simulink model "filterbank"  (R2018a)
settings: Solver=FixedStepDiscrete  StartTime=0.0  StopTime=inf  RelTol=1e-3
libraries: audiofilters x16, dspsrcs4 x2
settings Model: Creator=Kavi  LastModifiedBy=Kavi
settings SolverCC: AutoInsertRateTranBlk=on
settings DataIOCC: LimitDataPoints=on  SaveOutput=off  SignalLogging=off  SaveTime=off
settings OptimizationCC: LifeSpan=inf  SimCompilerOptimization=on
settings DebuggingCC: AlgebraicLoopMsg=error  SingleTaskRateTransMsg=error  AllowSymbolicDim=off  SFUnexpectedBacktrackingDiag=warning  SFNoUnconditionalDefaultTransitionDiag=warning  SFExecutionAtInitializationDiag=none
settings CodeAppCC: StateflowObjectComments=on
settings GRTTargetCC: TargetLangStandard=C89/C90 (ANSI)  GeneratePreprocessorConditionals=Disable all
settings ConfigComp: CovMetricSettings=dw  CovHtmlReporting=on  CovSaveCumulativeToWorkspaceVar=on  CovSaveSingleToWorkspaceVar=on  CovExternalEMLEnable=off  CovSFcnEnable=off

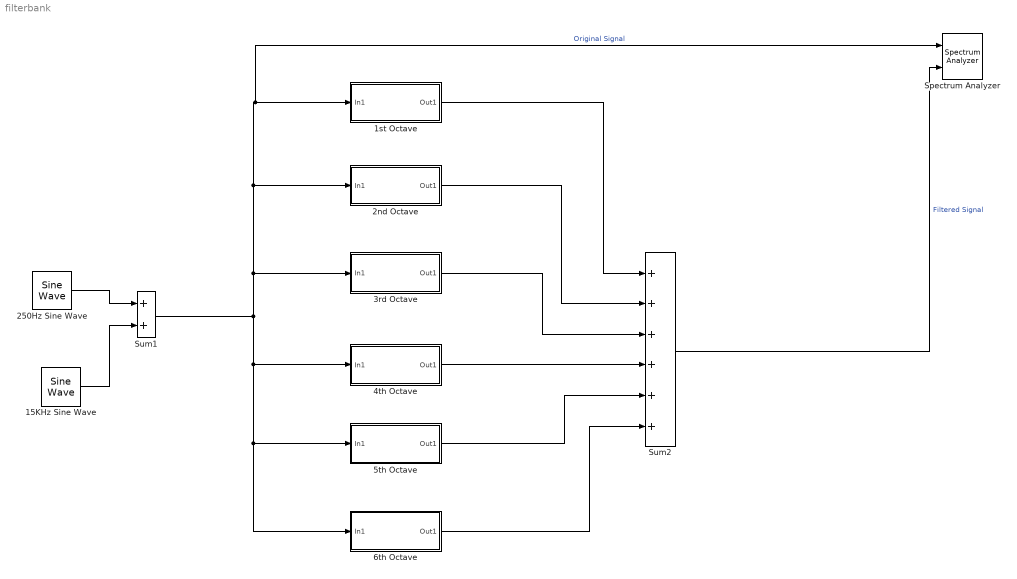
== system filterbank ==
  15KHz Sine Wave : dspsrcs4/Sine Wave  Amplitude=1  Frequency=314.98  Phase=0  SampleMode=Discrete  OutComplex=Real  CompMethod=Trigonometric fcn  TableSize=Speed  SampleTime=1/44100  SamplesPerFrame=256  ResetState=Restart at time zero  OutputFrames=off  dataType=double  wordLen=16  udDataType=sfix(16)  fracBitsMode=Best precision  numFracBits=15  OutDataTypeStr=double  LastOutDataTypeStr=double
  "1st Octave " : Subsystem
  250Hz Sine Wave : dspsrcs4/Sine Wave  Amplitude=1  Frequency=250  Phase=0  SampleMode=Discrete  OutComplex=Real  CompMethod=Trigonometric fcn  TableSize=Speed  SampleTime=1/44100  SamplesPerFrame=256  ResetState=Restart at time zero  OutputFrames=off  dataType=double  wordLen=16  udDataType=sfix(16)  fracBitsMode=Best precision  numFracBits=15  OutDataTypeStr=double  LastOutDataTypeStr=double
  2nd Octave : Subsystem
  "3rd Octave " : Subsystem
  4th Octave : Subsystem
  5th Octave : Subsystem
  6th Octave : Subsystem
  Spectrum Analyzer : SpectrumAnalyzer  NumInputPorts=2
  Sum1 : Sum
  Sum2 : Sum  Inputs=++++++
  wires:
  250Hz Sine Wave/1 -> Sum1/1
  15KHz Sine Wave/1 -> Sum1/2
  Sum1/1 -> "3rd Octave "/1(In1), "1st Octave "/1(In1), Spectrum Analyzer/1, 2nd Octave/1(In1), 6th Octave/1(In1), 5th Octave/1(In1), 4th Octave/1(In1)  "Original Signal"
  Sum2/1 -> Spectrum Analyzer/2  "Filtered Signal"
  2nd Octave/1(Out1) -> Sum2/2
  "3rd Octave "/1(Out1) -> Sum2/3
  4th Octave/1(Out1) -> Sum2/4
  5th Octave/1(Out1) -> Sum2/5
  6th Octave/1(Out1) -> Sum2/6
  "1st Octave "/1(Out1) -> Sum2/1

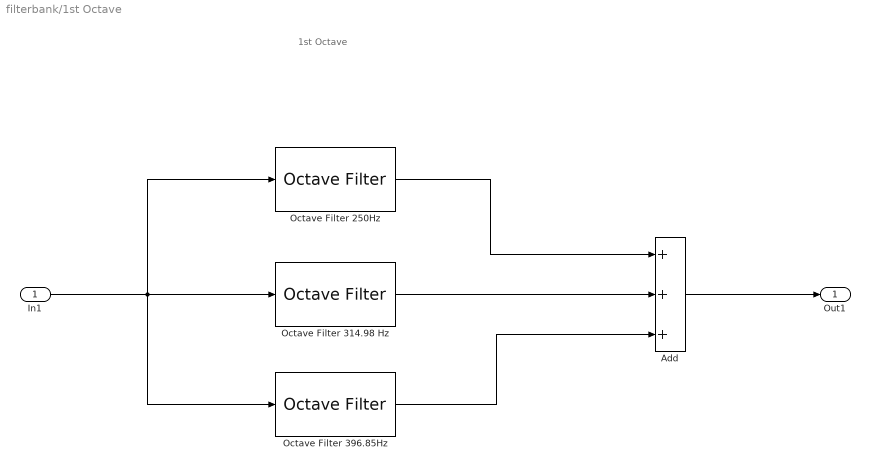
== system filterbank/1st Octave  ==
  note: 1st Octave
  In1 : Inport
  Add : Sum  Inputs=+++
  "Octave Filter 250Hz " : audiofilters/Octave Filter  FilterOrder=6  CenterFrequencyPort=off  CenterFrequency=250  Bandwidth=1 octave  BandsPerOctave=3  BandwidthType=1/3 octave  Oversample=off  InheritSampleRate=off  SampleRate=44100  SimulateUsing=Code generation  MaskClassType=Class 0
      settings: SourceProductName=Audio System Toolbox  SourceProductBaseCode=AU
  "Octave Filter 314.98 Hz " : audiofilters/Octave Filter  FilterOrder=6  CenterFrequencyPort=off  CenterFrequency=314.98  Bandwidth=1 octave  BandsPerOctave=3  BandwidthType=1/3 octave  Oversample=off  InheritSampleRate=off  SampleRate=44100  SimulateUsing=Code generation  MaskClassType=Class 0
      settings: SourceProductName=Audio System Toolbox  SourceProductBaseCode=AU
  "Octave Filter 396.85Hz " : audiofilters/Octave Filter  FilterOrder=6  CenterFrequencyPort=off  CenterFrequency=396.85  Bandwidth=1 octave  BandsPerOctave=3  BandwidthType=1/3 octave  Oversample=off  InheritSampleRate=off  SampleRate=44100  SimulateUsing=Code generation  MaskClassType=Class 0
      settings: SourceProductName=Audio System Toolbox  SourceProductBaseCode=AU
  Out1 : Outport
  wires:
  In1/1 -> "Octave Filter 250Hz "/1, "Octave Filter 314.98 Hz "/1, "Octave Filter 396.85Hz "/1
  "Octave Filter 314.98 Hz "/1 -> Add/2
  "Octave Filter 250Hz "/1 -> Add/1
  "Octave Filter 396.85Hz "/1 -> Add/3
  Add/1 -> Out1/1

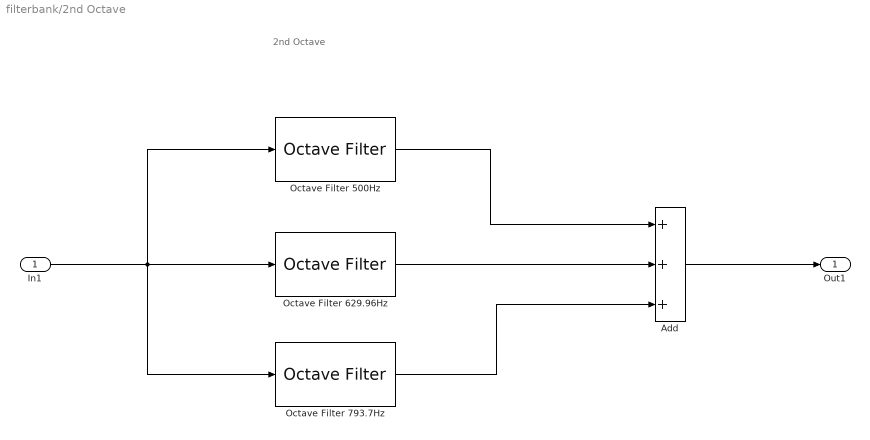
== system filterbank/2nd Octave ==
  note: 2nd Octave
  In1 : Inport
  Add : Sum  Inputs=+++
  "Octave Filter 500Hz " : audiofilters/Octave Filter  FilterOrder=6  CenterFrequencyPort=off  CenterFrequency=500  Bandwidth=1 octave  BandsPerOctave=3  BandwidthType=1/3 octave  Oversample=off  InheritSampleRate=off  SampleRate=44100  SimulateUsing=Code generation  MaskClassType=Class 0
      settings: SourceProductName=Audio System Toolbox  SourceProductBaseCode=AU
  "Octave Filter 629.96Hz " : audiofilters/Octave Filter  FilterOrder=6  CenterFrequencyPort=off  CenterFrequency=629.96  Bandwidth=1 octave  BandsPerOctave=3  BandwidthType=1/3 octave  Oversample=off  InheritSampleRate=off  SampleRate=44100  SimulateUsing=Code generation  MaskClassType=Class 0
      settings: SourceProductName=Audio System Toolbox  SourceProductBaseCode=AU
  "Octave Filter 793.7Hz " : audiofilters/Octave Filter  FilterOrder=6  CenterFrequencyPort=off  CenterFrequency=793.7  Bandwidth=1 octave  BandsPerOctave=3  BandwidthType=1/3 octave  Oversample=off  InheritSampleRate=off  SampleRate=44100  SimulateUsing=Code generation  MaskClassType=Class 0
      settings: SourceProductName=Audio System Toolbox  SourceProductBaseCode=AU
  Out1 : Outport
  wires:
  In1/1 -> "Octave Filter 500Hz "/1, "Octave Filter 629.96Hz "/1, "Octave Filter 793.7Hz "/1
  "Octave Filter 629.96Hz "/1 -> Add/2
  "Octave Filter 500Hz "/1 -> Add/1
  "Octave Filter 793.7Hz "/1 -> Add/3
  Add/1 -> Out1/1

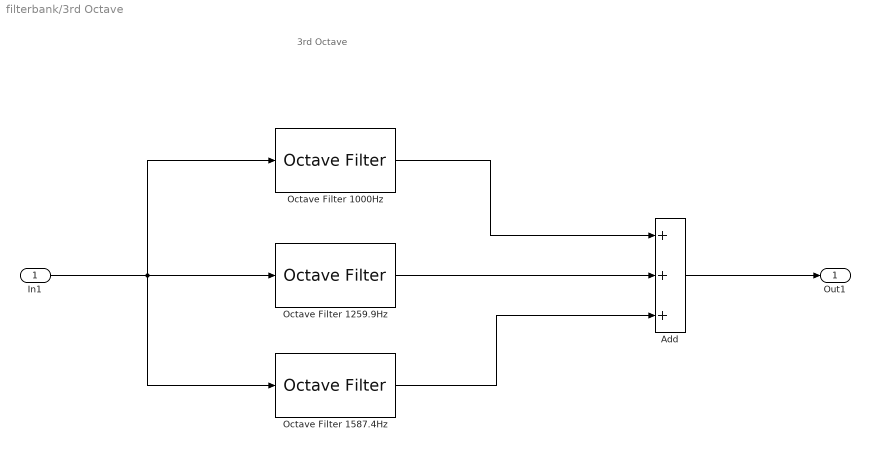
== system filterbank/3rd Octave  ==
  note: 3rd Octave
  In1 : Inport
  Add : Sum  Inputs=+++
  "Octave Filter 1000Hz " : audiofilters/Octave Filter  FilterOrder=6  CenterFrequencyPort=off  CenterFrequency=1000  Bandwidth=1 octave  BandsPerOctave=3  BandwidthType=1/3 octave  Oversample=off  InheritSampleRate=off  SampleRate=44100  SimulateUsing=Code generation  MaskClassType=Class 0
      settings: SourceProductName=Audio System Toolbox  SourceProductBaseCode=AU
  "Octave Filter 1259.9Hz " : audiofilters/Octave Filter  FilterOrder=6  CenterFrequencyPort=off  CenterFrequency=314.98  Bandwidth=1 octave  BandsPerOctave=3  BandwidthType=1/3 octave  Oversample=off  InheritSampleRate=off  SampleRate=44100  SimulateUsing=Code generation  MaskClassType=Class 0
      settings: SourceProductName=Audio System Toolbox  SourceProductBaseCode=AU
  "Octave Filter 1587.4Hz " : audiofilters/Octave Filter  FilterOrder=6  CenterFrequencyPort=off  CenterFrequency=1587.4  Bandwidth=1 octave  BandsPerOctave=3  BandwidthType=1/3 octave  Oversample=off  InheritSampleRate=off  SampleRate=44100  SimulateUsing=Code generation  MaskClassType=Class 0
      settings: SourceProductName=Audio System Toolbox  SourceProductBaseCode=AU
  Out1 : Outport
  wires:
  In1/1 -> "Octave Filter 1000Hz "/1, "Octave Filter 1259.9Hz "/1, "Octave Filter 1587.4Hz "/1
  "Octave Filter 1259.9Hz "/1 -> Add/2
  "Octave Filter 1000Hz "/1 -> Add/1
  "Octave Filter 1587.4Hz "/1 -> Add/3
  Add/1 -> Out1/1

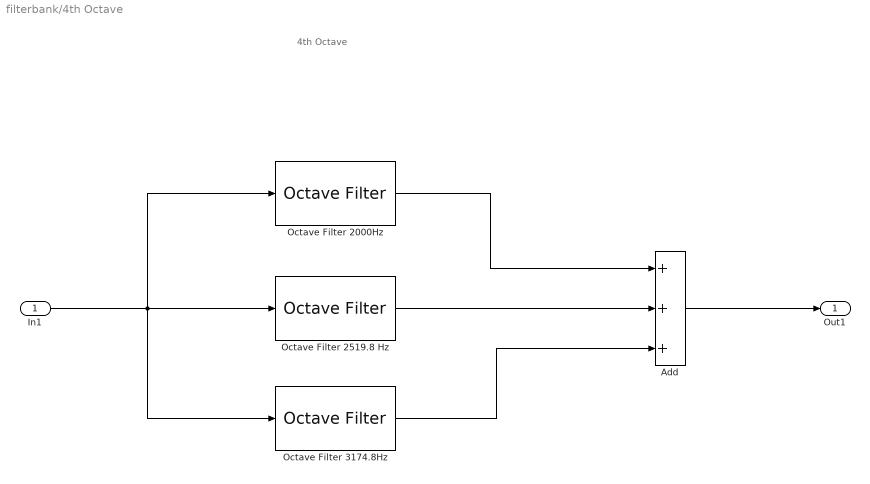
== system filterbank/4th Octave ==
  note: 4th Octave
  In1 : Inport
  Add : Sum  Inputs=+++
  "Octave Filter 2000Hz " : audiofilters/Octave Filter  FilterOrder=6  CenterFrequencyPort=off  CenterFrequency=2000  Bandwidth=1 octave  BandsPerOctave=3  BandwidthType=1/3 octave  Oversample=off  InheritSampleRate=off  SampleRate=44100  SimulateUsing=Code generation  MaskClassType=Class 0
      settings: SourceProductName=Audio System Toolbox  SourceProductBaseCode=AU
  "Octave Filter 2519.8 Hz " : audiofilters/Octave Filter  FilterOrder=6  CenterFrequencyPort=off  CenterFrequency=2519.8  Bandwidth=1 octave  BandsPerOctave=3  BandwidthType=1/3 octave  Oversample=off  InheritSampleRate=off  SampleRate=44100  SimulateUsing=Code generation  MaskClassType=Class 0
      settings: SourceProductName=Audio System Toolbox  SourceProductBaseCode=AU
  "Octave Filter 3174.8Hz " : audiofilters/Octave Filter  FilterOrder=6  CenterFrequencyPort=off  CenterFrequency=3174.8  Bandwidth=1 octave  BandsPerOctave=3  BandwidthType=1/3 octave  Oversample=off  InheritSampleRate=off  SampleRate=44100  SimulateUsing=Code generation  MaskClassType=Class 0
      settings: SourceProductName=Audio System Toolbox  SourceProductBaseCode=AU
  Out1 : Outport
  wires:
  In1/1 -> "Octave Filter 2000Hz "/1, "Octave Filter 2519.8 Hz "/1, "Octave Filter 3174.8Hz "/1
  "Octave Filter 2519.8 Hz "/1 -> Add/2
  "Octave Filter 2000Hz "/1 -> Add/1
  "Octave Filter 3174.8Hz "/1 -> Add/3
  Add/1 -> Out1/1

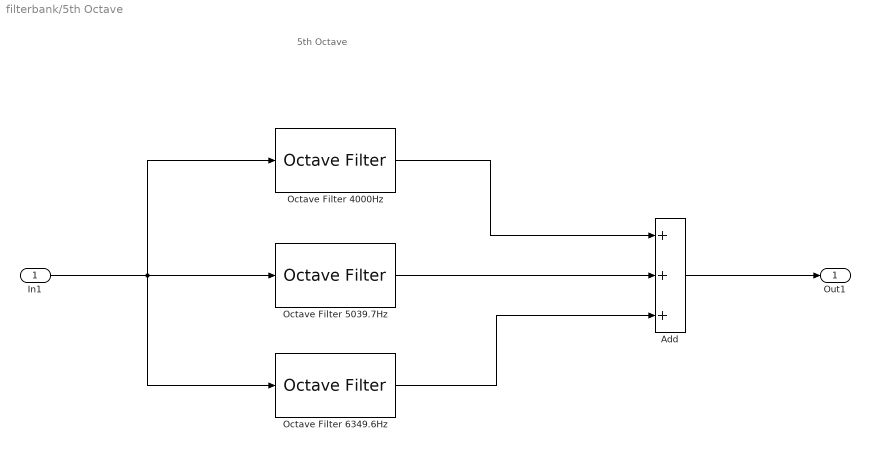
== system filterbank/5th Octave ==
  note: 5th Octave
  In1 : Inport
  Add : Sum  Inputs=+++
  "Octave Filter 4000Hz " : audiofilters/Octave Filter  FilterOrder=6  CenterFrequencyPort=off  CenterFrequency=4000  Bandwidth=1 octave  BandsPerOctave=3  BandwidthType=1/3 octave  Oversample=off  InheritSampleRate=off  SampleRate=44100  SimulateUsing=Code generation  MaskClassType=Class 0
      settings: SourceProductName=Audio System Toolbox  SourceProductBaseCode=AU
  "Octave Filter 5039.7Hz " : audiofilters/Octave Filter  FilterOrder=6  CenterFrequencyPort=off  CenterFrequency=5039.7  Bandwidth=1 octave  BandsPerOctave=3  BandwidthType=1/3 octave  Oversample=off  InheritSampleRate=off  SampleRate=44100  SimulateUsing=Code generation  MaskClassType=Class 0
      settings: SourceProductName=Audio System Toolbox  SourceProductBaseCode=AU
  "Octave Filter 6349.6Hz " : audiofilters/Octave Filter  FilterOrder=6  CenterFrequencyPort=off  CenterFrequency=6349.6  Bandwidth=1 octave  BandsPerOctave=3  BandwidthType=1/3 octave  Oversample=off  InheritSampleRate=off  SampleRate=44100  SimulateUsing=Code generation  MaskClassType=Class 0
      settings: SourceProductName=Audio System Toolbox  SourceProductBaseCode=AU
  Out1 : Outport
  wires:
  In1/1 -> "Octave Filter 4000Hz "/1, "Octave Filter 5039.7Hz "/1, "Octave Filter 6349.6Hz "/1
  "Octave Filter 5039.7Hz "/1 -> Add/2
  "Octave Filter 4000Hz "/1 -> Add/1
  "Octave Filter 6349.6Hz "/1 -> Add/3
  Add/1 -> Out1/1

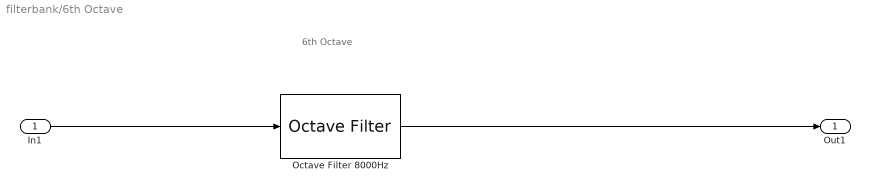
== system filterbank/6th Octave ==
  note: 6th Octave
  In1 : Inport
  "Octave Filter 8000Hz " : audiofilters/Octave Filter  FilterOrder=6  CenterFrequencyPort=off  CenterFrequency=8000  Bandwidth=1 octave  BandsPerOctave=3  BandwidthType=1/3 octave  Oversample=off  InheritSampleRate=off  SampleRate=44100  SimulateUsing=Code generation  MaskClassType=No mask
      settings: SourceProductName=Audio System Toolbox  SourceProductBaseCode=AU
  Out1 : Outport
  wires:
  In1/1 -> "Octave Filter 8000Hz "/1
  "Octave Filter 8000Hz "/1 -> Out1/1
